simulink model "four_to_four_switch_simulink"  (R2024b)
settings: Solver=VariableStepAuto  StartTime=0.0  StopTime=10.0  RelTol=1e-3
settings Model: Creator=samue  LastModifiedBy=samue
settings OptimizationCC: BlockReduction=off  ConditionallyExecuteInputs=off  DefaultParameterBehavior=Inlined
settings DebuggingCC: AlgebraicLoopMsg=error
settings HardwareCC: ProdBitPerPointer=32  ProdBitPerSizeT=32  ProdBitPerPtrDiffT=32  ProdLargestAtomicFloat=None  ProdIntDivRoundTo=Undefined  ProdEndianess=Unspecified  ProdWordSize=32  ProdHWDeviceType=ASIC/FPGA->ASIC/FPGA  TargetBitPerPointer=64  TargetBitPerSizeT=64  TargetBitPerPtrDiffT=64  TargetLongLongMode=on  TargetIntDivRoundTo=Zero  TargetEndianess=LittleEndian  TargetWordSize=64  TargetHWDeviceType=Custom Processor->MATLAB Host Computer  ProdEqTarget=off

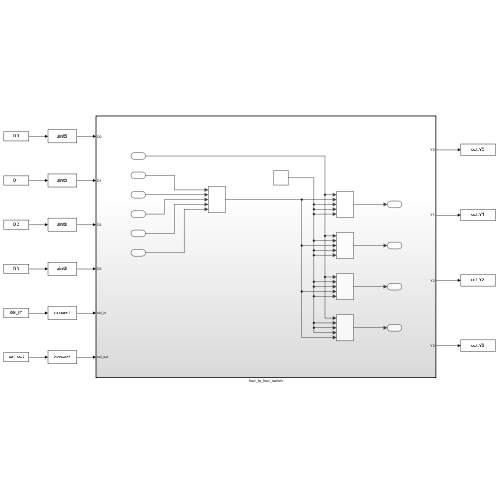
[thumbnail: Simulink's stored preview of the top-level diagram]
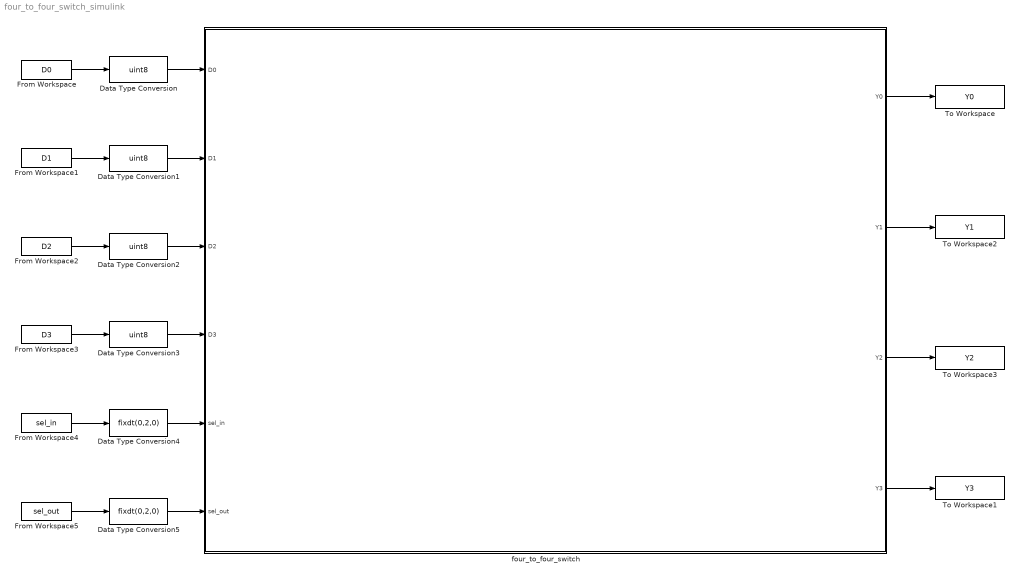
== system four_to_four_switch_simulink ==
  Data Type Conversion{,1..3} (4 alike) : DataTypeConversion  OutDataTypeStr=uint8  SaturateOnIntegerOverflow=off  RndMeth=Floor
  Data Type Conversion4 : DataTypeConversion  OutDataTypeStr=fixdt(0,2,0)  SaturateOnIntegerOverflow=off  RndMeth=Floor
  Data Type Conversion5 : DataTypeConversion  OutDataTypeStr=fixdt(0,2,0)  SaturateOnIntegerOverflow=off  RndMeth=Floor
  From Workspace : FromWorkspace  VariableName=D0  SampleTime=1
  From Workspace1 : FromWorkspace  VariableName=D1  SampleTime=1
  From Workspace2 : FromWorkspace  VariableName=D2  SampleTime=1
  From Workspace3 : FromWorkspace  VariableName=D3  SampleTime=1
  From Workspace4 : FromWorkspace  VariableName=sel_in  SampleTime=1
  From Workspace5 : FromWorkspace  VariableName=sel_out  SampleTime=1
  To Workspace : ToWorkspace  VariableName=Y0  SaveFormat=Timeseries  SampleTime=-1
  To Workspace1 : ToWorkspace  VariableName=Y3  SaveFormat=Timeseries  SampleTime=-1
  To Workspace2 : ToWorkspace  VariableName=Y1  SaveFormat=Timeseries  SampleTime=-1
  To Workspace3 : ToWorkspace  VariableName=Y2  SaveFormat=Timeseries  SampleTime=-1
  four_to_four_switch : Subsystem  TreatAsAtomicUnit=on
  wires:
  From Workspace/1 -> Data Type Conversion/1
  From Workspace5/1 -> Data Type Conversion5/1
  From Workspace1/1 -> Data Type Conversion1/1
  From Workspace2/1 -> Data Type Conversion2/1
  From Workspace4/1 -> Data Type Conversion4/1
  four_to_four_switch/4(Y3) -> To Workspace1/1
  From Workspace3/1 -> Data Type Conversion3/1
  four_to_four_switch/1(Y0) -> To Workspace/1
  four_to_four_switch/2(Y1) -> To Workspace2/1
  four_to_four_switch/3(Y2) -> To Workspace3/1
  Data Type Conversion/1 -> four_to_four_switch/1(D0)
  Data Type Conversion1/1 -> four_to_four_switch/2(D1)
  Data Type Conversion2/1 -> four_to_four_switch/3(D2)
  Data Type Conversion3/1 -> four_to_four_switch/4(D3)
  Data Type Conversion4/1 -> four_to_four_switch/5(sel_in)
  Data Type Conversion5/1 -> four_to_four_switch/6(sel_out)

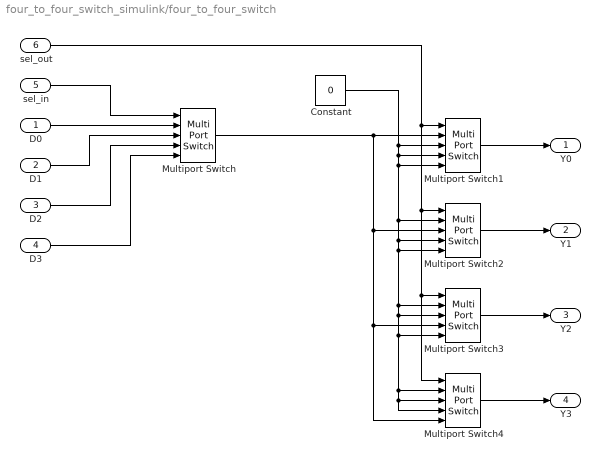
== system four_to_four_switch_simulink/four_to_four_switch ==
  D0 : Inport  OutDataTypeStr=uint8
  D1 : Inport  Port=2  OutDataTypeStr=uint8
  D2 : Inport  Port=3  OutDataTypeStr=uint8
  D3 : Inport  Port=4  OutDataTypeStr=uint8
  sel_in : Inport  Port=5  OutDataTypeStr=fixdt(0,2,0)
  sel_out : Inport  Port=6  OutDataTypeStr=fixdt(0,2,0)
  Constant : Constant  Value=0  OutDataTypeStr=uint8  SampleTime=-1
  Multiport Switch{,1..4} (5 alike) : MultiPortSwitch  DataPortOrder=Zero-based contiguous  Inputs=4  zeroidx=on  OutDataTypeStr=uint8  SaturateOnIntegerOverflow=off  InputSameDT=off
  Y0 : Outport  OutDataTypeStr=uint8  VectorParamsAs1DForOutWhenUnconnected=off
  Y1 : Outport  Port=2  OutDataTypeStr=uint8  VectorParamsAs1DForOutWhenUnconnected=off
  Y2 : Outport  Port=3  OutDataTypeStr=uint8  VectorParamsAs1DForOutWhenUnconnected=off
  Y3 : Outport  Port=4  OutDataTypeStr=uint8  VectorParamsAs1DForOutWhenUnconnected=off
  wires:
  sel_out/1 -> Multiport Switch4/1, Multiport Switch3/1, Multiport Switch2/1, Multiport Switch1/1
  Multiport Switch/1 -> Multiport Switch4/5, Multiport Switch3/4, Multiport Switch2/3, Multiport Switch1/2
  Constant/1 -> Multiport Switch4/4, Multiport Switch4/3, Multiport Switch4/2, Multiport Switch3/5, Multiport Switch3/3, Multiport Switch3/2, Multiport Switch2/5, Multiport Switch2/4, Multiport Switch2/2, Multiport Switch1/5, Multiport Switch1/4, Multiport Switch1/3
  sel_in/1 -> Multiport Switch/1
  D0/1 -> Multiport Switch/2
  D2/1 -> Multiport Switch/4
  Multiport Switch3/1 -> Y2/1
  Multiport Switch1/1 -> Y0/1
  D3/1 -> Multiport Switch/5
  Multiport Switch2/1 -> Y1/1
  D1/1 -> Multiport Switch/3
  Multiport Switch4/1 -> Y3/1
